simulink model "resp_test"  (R2016b)
settings: Solver=VariableStepAuto  StartTime=0.0  StopTime=60  RelTol=1e-3
values from neighbouring files (symbols this model uses):
  coef_a = 1    [MRAC_test.m]    (also in model_gen.m)
  coef_b = 2*zta*w_n    [MRAC_test.m]    (also in model_gen.m)
  coef_c = w_n^2    [MRAC_test.m]    (also in model_gen.m = w_n)
settings Model: Creator=CFreeman  LastModifiedBy=CFreeman

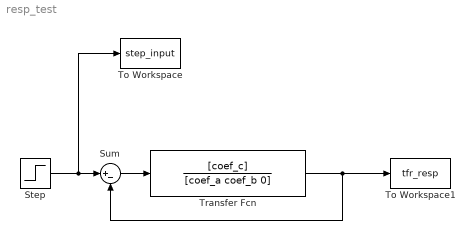
== system resp_test ==
  Step : Step  Time=5  After=20  SampleTime=0
  Sum : Sum  Inputs=|+-
  To Workspace : ToWorkspace  VariableName=step_input  SaveFormat=Timeseries  SampleTime=-1
  To Workspace1 : ToWorkspace  VariableName=tfr_resp  SaveFormat=Timeseries  SampleTime=-1
  Transfer Fcn : TransferFcn  Numerator=[coef_c]  Denominator=[coef_a coef_b 0]
  wires:
  Step/1 -> Sum/1, To Workspace/1
  Transfer Fcn/1 -> Sum/2, To Workspace1/1
  Sum/1 -> Transfer Fcn/1
